simulink model "OnBoardOk"  (R2015b)
settings: Solver=FixedStepDiscrete  SolverMode=SingleTasking  StartTime=0.0  StopTime=10.0  FixedStep=0.002  RelTol=1e-3
PreLoadFcn:
  | waijung.modelPreload; % Required for working with Waijung Blockset. Do not remove.
undefined symbols (not defined in the file): CPHA_1Edge, CPOL_Low, Duplex, FirstBit_MSB, Full, Link, LQFP100, ST, STM32F407VG, STM32F4DISCOVERY
libraries: simulink x12, stm32f4_io_lib x5, stm32f4_spi_lib x3, stm32f4_device_config_lib x1, BC_USB x1, stm32f4_adc_lib x1
(part 1 of 2)
CloseFcn:
  | waijung.modelClose; % Required for working with Waijung Blockset. Do not remove.
settings Model: Creator=Hi  LastModifiedBy=Jasper Gundersen
settings DataIOCC: SaveFormat=Array
settings OptimizationCC: OptimizeModelRefInitCode=on  LifeSpan=1
settings HardwareCC: ProdBitPerPointer=32  ProdLargestAtomicFloat=None  ProdIntDivRoundTo=Undefined  ProdWordSize=32  ProdHWDeviceType=ARM Compatible->Cortex - M4  TargetEndianess=LittleEndian  TargetHWDeviceType=ARM Compatible->Cortex - M4
settings RTWCC: SystemTargetFile=stm32f4.tlc  GenerateMakefile=off  TemplateMakefile=ert_default_tmf  Description=STM32F4 Target
settings CodeAppCC: ForceParamTrailComments=on  IgnoreCustomStorageClasses=off  OperatorAnnotations=on  SimulinkDataObjDesc=on  InsertBlockDesc=on  MATLABSourceComments=on
settings STFCustomTargetCC: ModelReferenceCompliant=off  ConcurrentExecutionCompliant=off  GeneratePreprocessorConditionals=Use local settings  CombineOutputUpdateFcns=on  ERTCustomFileBanners=on  SupportContinuousTime=off  SupportNonInlinedSFcns=off  MATLABClassNameForMDSCustomization=Simulink.SoftwareTarget.ERTCustomization  CPPClassGenCompliant=off  GRTInterface=off  SystemTargetFile=stm32f4.tlc
settings ERTTargetCC: ModelReferenceCompliant=off  ParMdlRefBuildCompliant=off  CompOptLevelCompliant=off  ConcurrentExecutionCompliant=off  ERTFirstTimeCompliant=off  ModelStepFunctionPrototypeControlCompliant=off  CPPClassGenCompliant=off  UseToolchainInfoCompliant=off  ERTSrcFileBannerTemplate=stm32f4_code_template.cgt  ERTHdrFileBannerTemplate=stm32f4_code_template.cgt  ERTDataSrcFileTemplate=stm32f4_code_template.cgt  ERTDataHdrFileTemplate=stm32f4_code_template.cgt  ERTCustomFileTemplate=stm32f4_file_process.tlc
settings ConfigComp: CovModelRefEnable=Off

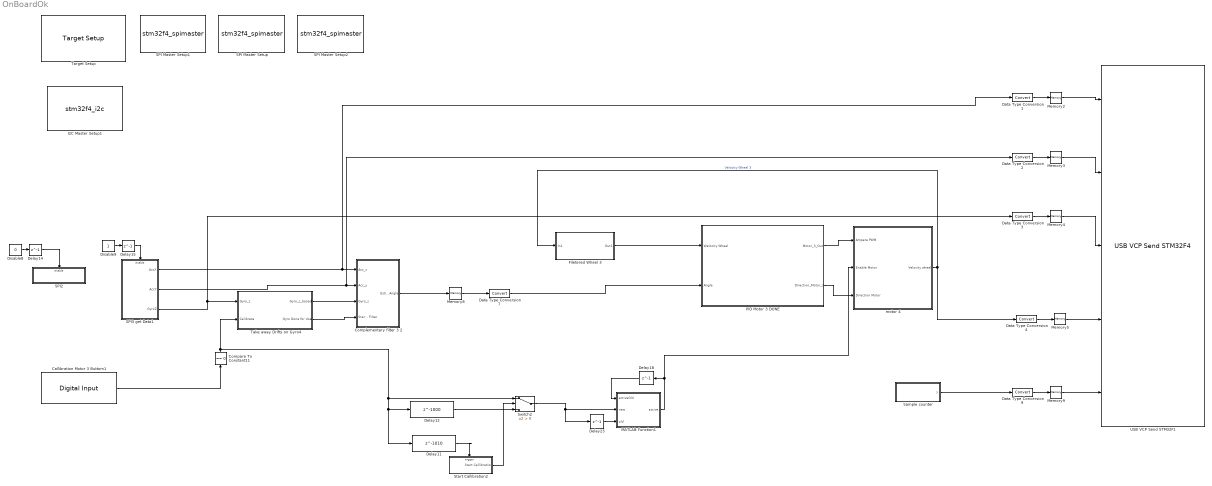
== system OnBoardOk ==
  Callibration Motor 3 Buttom1 : stm32f4_io_lib/Digital Input  port=E  speed=100  porttype=Pull Up  porttypestr=UP  use_pin0=off  use_pin1=off  use_pin2=off  use_pin3=off  use_pin4=off  use_pin5=off  use_pin6=off  use_pin7=off  use_pin8=off  use_pin9=off  use_pin10=on  use_pin11=off  use_pin12=off  use_pin13=off  use_pin14=off  use_pin15=off  pinstr=GPIO_Pin_10  usedpinarray="[0  0  0  0  0  0  0  0  0  0  1  0  0  0  0  0]"  bitbandingstr="#define CallibrationMotor3Buttom1_E10 Peripheral_BB(GPIOE->IDR, 10)  /* Output pin */"  sampletime=0.002  sampletimestr=0.002  blockid=CallibrationMotor3Buttom1  enablecustomportlabel=off  glabalinit=off  cinputportlabel=In1, In2  coutputportlabel=Out1, Out2
  Compare To Constant11 : simulink/Logic and Bit Operations/Compare To Constant  relop===  const=0  OutDataTypeStr=boolean  ZeroCross=off
  Complementary filter 3 2 : Subsystem
  Data Type Conversion{1..4,7,9} (6 alike) : DataTypeConversion
  Delay11 : Delay  DelayLength=1010  InitialCondition=0
  Delay12 : Delay  DelayLength=1000  InitialCondition=0
  Delay14 : Delay  DelayLength=1  InitialCondition=1
  Delay15 : Delay  DelayLength=1  InitialCondition=0
  Delay18 : Delay  DelayLength=1  InitialCondition=0
  Delay23 : Delay  DelayLength=1  InitialCondition=0
  Disable8 : Constant  Value=0
  Disable9 : Constant
  Filetered Wheel 3 : Subsystem
  I2C Master Setup1 : S-Function  FunctionName=stm32f4_i2c  Parameters=configuration,module,transfer,clkspeed,timeout,sdapin,sclpin,writecount,readcount,inputtypearray,outputtypearray,confstr,sampletime,sampletimestr,blockid  SFunctionDeploymentMode=off  EnableBusSupport=off  mask(stm32f4_i2c){configuration=Setup, module=1, lastmodule=1, transfer=Blocking, dutycycle=TLow/THigh = 2, clkspeed=400, timeout=25, writecount=0, readcount=0, sdapin=B7, sclpin=B6, waitwritetime=0, inputtypearray=[0], outputtypearray=[0], confstr=["B","7","B","6","1","1","6","0","I2C_DutyCycle_2","0","off"], sampletime=-1, sampletimestr=0.002, blockid=I2CMasterSetup1}
      mask prompts: module "I2C Module"; lastmodule "Last module"; transfer "Transfer mode"; dutycycle "Duty cycle in fast mode"; clkspeed "Clock speed (kHz)"; timeout "Timeout (ms)"; writecount "Bytes write count"; readcount "Bytes read count"; sdapin "SDA pin"; sclpin "SCL pin"; waitwritetime "Wait write time (ms), default is 0"; inputtypearray "Input type array"; outputtypearray "Output type array"; confstr "Configuration string"; sampletime "Sample time (sec)"; sampletimestr "Compiled sample time (sec) in string"
      mask init:
      | stm32f4_i2c_callback('init');
      mask Help: web(fullfile(waijungdocroot,'stm32f4_i2c_setup.htm'), '-browser')
      mask TypeOptions configuration: Setup | Transaction
      mask Callback configuration: stm32f4_i2c_callback('configuration');
      mask TypeOptions module: 1 | 2 | 3
      mask Callback module: stm32f4_i2c_callback('module');
      mask TypeOptions transfer: Blocking | Non-blocking
      mask TypeOptions dutycycle: TLow/THigh = 16/9 | TLow/THigh = 2
      mask Callback dutycycle: stm32f4_i2c_callback('dutycycle');
      mask Callback writecount: stm32f4_i2c_callback('writecount');
      mask Callback readcount: stm32f4_i2c_callback('readcount');
      mask TypeOptions sdapin: - | B7 | B9
      mask Callback sdapin: stm32f4_i2c_callback('sdapin');
      mask TypeOptions sclpin: - | B6 | B8
      mask Callback sclpin: stm32f4_i2c_callback('sclpin');
      mask Callback confstr: stm32f4_i2c_callback('confstr');
      mask Callback sampletime: stm32f4_i2c_callback('sampletime');
      mask Callback sampletimestr: stm32f4_i2c_callback('sampletimestr');
      mask Callback blockid: stm32f4_i2c_callback('blockid');
      mask Display: text(0.5, 0.5, 'Module: I2C1\nClock: 400kHz\nSDA/SCL Pin: B7/B6','ver','middle','hor','center');
  MATLAB Function1 : MATLAB Function  TreatAsAtomicUnit=on
  Memory{2..5,8..9} (6 alike) : Memory  InheritSampleTime=on
  "PID Motor 3 DONE " : Subsystem
  SPI Master Setup : S-Function  FunctionName=stm32f4_spimaster  Parameters=mode,configuration,module,datacount,inputtypearray,outputtypearray,confstr,sampletime,sampletimestr,blockid  SFunctionDeploymentMode=off  EnableBusSupport=off  mask(stm32f4_spimaster){configuration=Setup, module=2, mode=Write, lastmodule=2, direction=Full-Duplex, dataformat=8bit/ FirstBit_MSB, prescaler=32, lastpclk=42000000, baudrate=1312500, cpolcpha=CPOL_Low/ CPHA_1Edge, datacount=0, nssmode=Software, nsspin=Not used, softnssport=B, softnsspin=12, sckpin=B13, misopin=B14, mosipin=B15, pintype=Push Pull, pulltype=Pull Up, nssdelay=0, inputtypearray=[0], outputtypearray=[0], confstr=["SPI_Direction_2Lines_FullDuplex","8b","MSB","Low","1Edge","32","Soft","0","x","x","1","B","12","1","B","13","1","B","14","1","B","15","0","1","0","0","0","0","0","0","0","PP","0","UP"], sampletime=-1, sampletimestr=0.002, blockid=SPIMasterSetup}
      mask prompts: module "SPI Module:"; lastmodule "Last module:"; dataformat "Data format:"; prescaler "Buad rate prescaler: Pclk/"; lastpclk "Last PCLK"; baudrate "Baud rate (Hz)"; cpolcpha "Clock polarity (CPOL)/ Clock phase (CPHA):"; datacount "Data Write count:"; nssmode "Slave/chip select (nSS, nCS) mode"; nsspin "Slave/chip select (nSS, nCS) pin"; softnssport "Slave/chip select port (nSS, nCS)"; softnsspin "Slave/chip select pin (nSS, nCS)"; sckpin "SCLK pin:"; misopin "MISO pin:"; mosipin "MOSI pin:"; pintype "Pin type (Push-Pull/Open-Drain)"; pulltype "Pull Type (Up/Down)"; nssdelay "Data delay time, uS:"; inputtypearray "Input type array"; outputtypearray "Output type array"; confstr "Configuration string"; sampletime "Sample time (sec)"; sampletimestr "Compiled sample time (sec) in string"
      mask help:
      | Direction:
      |  - Full-Duplex, use this mode when need to send and receive data at same clock.
      |  - Half-Duplex_Tx, this mode is to transmit data to slave only. Pin MISO (Rx) can be free for other function.
      |  - Half-Duplex_Rx, this mode is to receive data from slave only. Pin MOSIO (Tx) can be free for other function.
      | Data format:
      |   This configuration is depending on the specification of slave device.
      | Baud rate prescaler:
      |  - Use this prescaler to devide from the PCLK for SPI clock.
      |  - This Prescaler value is auto determine corresponding to baudrate setting and selected SPI module.
      | Baud rate (Hz):
      |  - Select baud rate for SPI clock. Please check the maximum clock support for target slave device.
      | Clock polarity and Clock phase:
      |  - This configuration parameter is depending on slave device.
      |  - See waijung help for more description.
      | Slave/chip select mode:
      |  - Hardware, use hardware SPI module for slave select (or chip select) pin.
      |  - Software, this mode allow any available pin for slave select (or chip select) function.
      |  - Custom, SPI block did not control slave select pin. User may use Digital Output block to control by costom.
      mask init:
      | stm32f4_spimaster_callback('init');
      mask Help: web(fullfile(waijungdocroot,'stm32f4_spimaster_setup.htm'), '-browser')
      mask TypeOptions configuration: Setup | Transaction
      mask Callback configuration: stm32f4_spimaster_callback('configuration');
      mask TypeOptions module: 1 | 2 | 3
      mask Callback module: stm32f4_spimaster_callback('module');
      mask TypeOptions mode: Read/ Write | Read | Write
      mask Callback mode: stm32f4_spimaster_callback('mode');
      mask TypeOptions direction: Full-Duplex | Half-Duplex_Tx | Half-Duplex_Rx
      mask Callback direction: stm32f4_spimaster_callback('direction');
      mask TypeOptions dataformat: 8bit/ FirstBit_MSB | 8bit/ FirstBit_LSB | 16bit/ FirstBit_MSB | 16bit/ FirstBit_LSB
      mask TypeOptions prescaler: 2 | 4 | 8 | 16 | 32 | 64 | 128 | 256
      mask TypeOptions baudrate: Not set | 21000000 | 10500000 | 5250000 | 2625000 | 1312500 | 656250 | 328125 | 164063
      mask Callback baudrate: stm32f4_spimaster_callback('baudrate');
      mask TypeOptions cpolcpha: CPOL_Low/ CPHA_1Edge | CPOL_Low/ CPHA_2Edge | CPOL_High/ CPHA_1Edge | CPOL_High/ CPHA_2Edge
      mask Callback datacount: stm32f4_spimaster_callback('datacount');
      mask TypeOptions nssmode: Hardware | Software | Custom
      mask Callback nssmode: stm32f4_spimaster_callback('nssmode');
      mask TypeOptions nsspin: Not used | B9 | B12
      mask TypeOptions softnssport: A | B | C | D | E | F | G | H | I
      mask TypeOptions softnsspin: 0 | 1 | 2 | 3 | 4 | 5 | 6 | 7 | 8 | 9 | 10 | 11 | 12 | 13 | 14 | 15
      mask TypeOptions sckpin: Not used | B10 | B13
      mask TypeOptions misopin: Not used | B14 | C2
      mask TypeOptions mosipin: Not used | B15 | C3
      mask TypeOptions pintype: Push Pull | Open Drain
      mask TypeOptions pulltype: None | Pull Up | Pull Down
      mask Callback confstr: stm32f4_spimaster_callback('confstr');
      mask Callback sampletime: stm32f4_spimaster_callback('sampletime');
      mask Callback sampletimestr: stm32f4_spimaster_callback('sampletimestr');
      mask Callback blockid: stm32f4_spimaster_callback('blockid');
      mask Display: text(0.5, 0.5, 'Module: SPI2 (Master)\nFull-Duplex\nBaudrate: 1312500','ver','middle','hor','center');
  SPI Master Setup1 : S-Function  FunctionName=stm32f4_spimaster  Parameters=mode,configuration,module,datacount,inputtypearray,outputtypearray,confstr,sampletime,sampletimestr,blockid  SFunctionDeploymentMode=off  EnableBusSupport=off  mask(stm32f4_spimaster){configuration=Setup, module=1, mode=Write, lastmodule=1, direction=Full-Duplex, dataformat=8bit/ FirstBit_MSB, prescaler=64, lastpclk=84000000, baudrate=1312500, cpolcpha=CPOL_Low/ CPHA_1Edge, datacount=0, nssmode=Software, nsspin=Not used, softnssport=C, softnsspin=5, sckpin=A5, misopin=A6, mosipin=A7, pintype=Push Pull, pulltype=Pull Up, nssdelay=0, inputtypearray=[0], outputtypearray=[0], confstr=["SPI_Direction_2Lines_FullDuplex","8b","MSB","Low","1Edge","64","Soft","0","x","x","1","C","5","1","A","5","1","A","6","1","A","7","1","0","1","0","0","0","0","0","0","PP","0","UP"], sampletime=-1, sampletimestr=0.002, blockid=SPIMasterSetup1}
      mask prompts: module "SPI Module:"; lastmodule "Last module:"; dataformat "Data format:"; prescaler "Buad rate prescaler: Pclk/"; lastpclk "Last PCLK"; baudrate "Baud rate (Hz)"; cpolcpha "Clock polarity (CPOL)/ Clock phase (CPHA):"; datacount "Data Write count:"; nssmode "Slave/chip select (nSS, nCS) mode"; nsspin "Slave/chip select (nSS, nCS) pin"; softnssport "Slave/chip select port (nSS, nCS)"; softnsspin "Slave/chip select pin (nSS, nCS)"; sckpin "SCLK pin:"; misopin "MISO pin:"; mosipin "MOSI pin:"; pintype "Pin type (Push-Pull/Open-Drain)"; pulltype "Pull Type (Up/Down)"; nssdelay "Data delay time, uS:"; inputtypearray "Input type array"; outputtypearray "Output type array"; confstr "Configuration string"; sampletime "Sample time (sec)"; sampletimestr "Compiled sample time (sec) in string"
      mask help:
      | Direction:
      |  - Full-Duplex, use this mode when need to send and receive data at same clock.
      |  - Half-Duplex_Tx, this mode is to transmit data to slave only. Pin MISO (Rx) can be free for other function.
      |  - Half-Duplex_Rx, this mode is to receive data from slave only. Pin MOSIO (Tx) can be free for other function.
      | Data format:
      |   This configuration is depending on the specification of slave device.
      | Baud rate prescaler:
      |  - Use this prescaler to devide from the PCLK for SPI clock.
      |  - This Prescaler value is auto determine corresponding to baudrate setting and selected SPI module.
      | Baud rate (Hz):
      |  - Select baud rate for SPI clock. Please check the maximum clock support for target slave device.
      | Clock polarity and Clock phase:
      |  - This configuration parameter is depending on slave device.
      |  - See waijung help for more description.
      | Slave/chip select mode:
      |  - Hardware, use hardware SPI module for slave select (or chip select) pin.
      |  - Software, this mode allow any available pin for slave select (or chip select) function.
      |  - Custom, SPI block did not control slave select pin. User may use Digital Output block to control by costom.
      mask init:
      | stm32f4_spimaster_callback('init');
      mask Help: web(fullfile(waijungdocroot,'stm32f4_spimaster_setup.htm'), '-browser')
      mask TypeOptions configuration: Setup | Transaction
      mask Callback configuration: stm32f4_spimaster_callback('configuration');
      mask TypeOptions module: 1 | 2 | 3
      mask Callback module: stm32f4_spimaster_callback('module');
      mask TypeOptions mode: Read/ Write | Read | Write
      mask Callback mode: stm32f4_spimaster_callback('mode');
      mask TypeOptions direction: Full-Duplex | Half-Duplex_Tx | Half-Duplex_Rx
      mask Callback direction: stm32f4_spimaster_callback('direction');
      mask TypeOptions dataformat: 8bit/ FirstBit_MSB | 8bit/ FirstBit_LSB | 16bit/ FirstBit_MSB | 16bit/ FirstBit_LSB
      mask TypeOptions prescaler: 2 | 4 | 8 | 16 | 32 | 64 | 128 | 256
      mask TypeOptions baudrate: Not set | 42000000 | 21000000 | 10500000 | 5250000 | 2625000 | 1312500 | 656250 | 328125
      mask Callback baudrate: stm32f4_spimaster_callback('baudrate');
      mask TypeOptions cpolcpha: CPOL_Low/ CPHA_1Edge | CPOL_Low/ CPHA_2Edge | CPOL_High/ CPHA_1Edge | CPOL_High/ CPHA_2Edge
      mask Callback datacount: stm32f4_spimaster_callback('datacount');
      mask TypeOptions nssmode: Hardware | Software | Custom
      mask Callback nssmode: stm32f4_spimaster_callback('nssmode');
      mask TypeOptions nsspin: Not used | A4 | A15
      mask TypeOptions softnssport: A | B | C | D | E | F | G | H | I
      mask TypeOptions softnsspin: 0 | 1 | 2 | 3 | 4 | 5 | 6 | 7 | 8 | 9 | 10 | 11 | 12 | 13 | 14 | 15
      mask TypeOptions sckpin: Not used | A5 | B3
      mask TypeOptions misopin: Not used | A6 | B4
      mask TypeOptions mosipin: Not used | A7 | B5
      mask TypeOptions pintype: Push Pull | Open Drain
      mask TypeOptions pulltype: None | Pull Up | Pull Down
      mask Callback confstr: stm32f4_spimaster_callback('confstr');
      mask Callback sampletime: stm32f4_spimaster_callback('sampletime');
      mask Callback sampletimestr: stm32f4_spimaster_callback('sampletimestr');
      mask Callback blockid: stm32f4_spimaster_callback('blockid');
      mask Display: text(0.5, 0.5, 'Module: SPI1 (Master)\nFull-Duplex\nBaudrate: 1312500','ver','middle','hor','center');
  SPI Master Setup2 : S-Function  FunctionName=stm32f4_spimaster  Parameters=mode,configuration,module,datacount,inputtypearray,outputtypearray,confstr,sampletime,sampletimestr,blockid  SFunctionDeploymentMode=off  EnableBusSupport=off  mask(stm32f4_spimaster){configuration=Setup, module=3, mode=Write, lastmodule=3, direction=Full-Duplex, dataformat=8bit/ FirstBit_MSB, prescaler=32, lastpclk=42000000, baudrate=1312500, cpolcpha=CPOL_Low/ CPHA_1Edge, datacount=0, nssmode=Software, nsspin=Not used, softnssport=C, softnsspin=11, sckpin=C10, misopin=B4, mosipin=B5, pintype=Push Pull, pulltype=Pull Up, nssdelay=0, inputtypearray=[0], outputtypearray=[0], confstr=["SPI_Direction_2Lines_FullDuplex","8b","MSB","Low","1Edge","32","Soft","0","x","x","1","C","11","1","C","10","1","B","4","1","B","5","0","1","1","0","0","0","0","0","0","PP","0","UP"], sampletime=-1, sampletimestr=0.002, blockid=SPIMasterSetup2}
      mask prompts: module "SPI Module:"; lastmodule "Last module:"; dataformat "Data format:"; prescaler "Buad rate prescaler: Pclk/"; lastpclk "Last PCLK"; baudrate "Baud rate (Hz)"; cpolcpha "Clock polarity (CPOL)/ Clock phase (CPHA):"; datacount "Data Write count:"; nssmode "Slave/chip select (nSS, nCS) mode"; nsspin "Slave/chip select (nSS, nCS) pin"; softnssport "Slave/chip select port (nSS, nCS)"; softnsspin "Slave/chip select pin (nSS, nCS)"; sckpin "SCLK pin:"; misopin "MISO pin:"; mosipin "MOSI pin:"; pintype "Pin type (Push-Pull/Open-Drain)"; pulltype "Pull Type (Up/Down)"; nssdelay "Data delay time, uS:"; inputtypearray "Input type array"; outputtypearray "Output type array"; confstr "Configuration string"; sampletime "Sample time (sec)"; sampletimestr "Compiled sample time (sec) in string"
      mask help:
      | Direction:
      |  - Full-Duplex, use this mode when need to send and receive data at same clock.
      |  - Half-Duplex_Tx, this mode is to transmit data to slave only. Pin MISO (Rx) can be free for other function.
      |  - Half-Duplex_Rx, this mode is to receive data from slave only. Pin MOSIO (Tx) can be free for other function.
      | Data format:
      |   This configuration is depending on the specification of slave device.
      | Baud rate prescaler:
      |  - Use this prescaler to devide from the PCLK for SPI clock.
      |  - This Prescaler value is auto determine corresponding to baudrate setting and selected SPI module.
      | Baud rate (Hz):
      |  - Select baud rate for SPI clock. Please check the maximum clock support for target slave device.
      | Clock polarity and Clock phase:
      |  - This configuration parameter is depending on slave device.
      |  - See waijung help for more description.
      | Slave/chip select mode:
      |  - Hardware, use hardware SPI module for slave select (or chip select) pin.
      |  - Software, this mode allow any available pin for slave select (or chip select) function.
      |  - Custom, SPI block did not control slave select pin. User may use Digital Output block to control by costom.
      mask init:
      | stm32f4_spimaster_callback('init');
      mask Help: web(fullfile(waijungdocroot,'stm32f4_spimaster_setup.htm'), '-browser')
      mask TypeOptions configuration: Setup | Transaction
      mask Callback configuration: stm32f4_spimaster_callback('configuration');
      mask TypeOptions module: 1 | 2 | 3
      mask Callback module: stm32f4_spimaster_callback('module');
      mask TypeOptions mode: Read/ Write | Read | Write
      mask Callback mode: stm32f4_spimaster_callback('mode');
      mask TypeOptions direction: Full-Duplex | Half-Duplex_Tx | Half-Duplex_Rx
      mask Callback direction: stm32f4_spimaster_callback('direction');
      mask TypeOptions dataformat: 8bit/ FirstBit_MSB | 8bit/ FirstBit_LSB | 16bit/ FirstBit_MSB | 16bit/ FirstBit_LSB
      mask TypeOptions prescaler: 2 | 4 | 8 | 16 | 32 | 64 | 128 | 256
      mask TypeOptions baudrate: Not set | 21000000 | 10500000 | 5250000 | 2625000 | 1312500 | 656250 | 328125 | 164063
      mask Callback baudrate: stm32f4_spimaster_callback('baudrate');
      mask TypeOptions cpolcpha: CPOL_Low/ CPHA_1Edge | CPOL_Low/ CPHA_2Edge | CPOL_High/ CPHA_1Edge | CPOL_High/ CPHA_2Edge
      mask Callback datacount: stm32f4_spimaster_callback('datacount');
      mask TypeOptions nssmode: Hardware | Software | Custom
      mask Callback nssmode: stm32f4_spimaster_callback('nssmode');
      mask TypeOptions nsspin: Not used | A4 | A15
      mask TypeOptions softnssport: A | B | C | D | E | F | G | H | I
      mask TypeOptions softnsspin: 0 | 1 | 2 | 3 | 4 | 5 | 6 | 7 | 8 | 9 | 10 | 11 | 12 | 13 | 14 | 15
      mask TypeOptions sckpin: Not used | B3 | C10
      mask TypeOptions misopin: Not used | B4 | C11
      mask TypeOptions mosipin: Not used | B5 | C12
      mask TypeOptions pintype: Push Pull | Open Drain
      mask TypeOptions pulltype: None | Pull Up | Pull Down
      mask Callback confstr: stm32f4_spimaster_callback('confstr');
      mask Callback sampletime: stm32f4_spimaster_callback('sampletime');
      mask Callback sampletimestr: stm32f4_spimaster_callback('sampletimestr');
      mask Callback blockid: stm32f4_spimaster_callback('blockid');
      mask Display: text(0.5, 0.5, 'Module: SPI3 (Master)\nFull-Duplex\nBaudrate: 1312500','ver','middle','hor','center');
  SPI2 : Subsystem  Priority=0  TreatAsAtomicUnit=on
  SPI3 get Data1 : Subsystem
  Sample counter : MATLAB Function  TreatAsAtomicUnit=on
  Start Callibration2 : Subsystem
  Switch2 : Switch  Criteria=u2 > Threshold
  Take away Drifts on Gyro4 : Subsystem
  Target Setup : stm32f4_device_config_lib/Target Setup  Priority=100  compiler=GNU ARM  previous_compiler=GNU ARM  mcu=STM32F407VG (LQFP100); STM32F4DISCOVERY  mcustr=STM32F407VG  clockconfig=STM32F4DISCOVERY Default (HSEOSC-8MHz/HCLK-168MHz)  system_stm32f4xx_c_path=C:\Users\Jasper Gundersen\Documents\Cube\waijung15_04a\targets\stm32f4_target\stm32f4\utils\STM32F4xx_AN3988_V1.0.1\stm32f4_default\hseosc8mhz  showmemoryconfiguration=off  stacksize=0x400  heapsize=0x200  enableautocompiledownload=on  fullchiperase=off  programmerinterface=ST-Link  editctrlstr=on  compilercontrolstr=$(patsubst %, -I%, .) -mcpu=cortex-m4 -mthumb -mthumb-interwork -mfloat-abi=hard -mfpu=fpv4-sp-d16 -ffast-math -Wall -Wextra -Ofast  assemblercontrolstr=$(patsubst %, -I%, .) -mcpu=cortex-m4 -mthumb -mthumb-interwork -mfloat-abi=hard -mfpu=fpv4-sp-d16 -ffast-math -Wall -Wextra -Ofast -Wa,-amhls=$(<:.s=.lst) -D__STACK_SIZE=$(STACK_SIZE) -D__HEAP_SIZE=$(HEAP_SIZE)  linkercontrolstr=-T$(LD_SCRIPT) -g -Wl,-Map=$(MAP),--cref,--no-warn-mismatch -mcpu=cortex-m4 -mthumb -mthumb-interwork -mfloat-abi=hard -mfpu=fpv4-sp-d16  runafterdownload=on  execprofile=None  profileruart=1  profilerbaud=115200  profilertxpin=Not used  profilerinitstr=0.002,168000000,336000,115200,0  manualsetsampletime=on  sampletime=0.002  blockid=TargetSetup  systickreloadvalue=336000  hseval=8000000  lastprofileruart=1  hclk=168000000  flashorigin=0x8000000  flashlength=1M  ramorigin=0x20000000  ramlength=112k  useextram=off
  USB VCP Send STM32F1 : BC_USB/USB VCP Send STM32F4  speed="USB 1.1   12Mbit/s"  data_size=2048 Bytes  header_data='0E 0E'  binary_data='double double double double double'  terminator_data='0A 0A'  sampletime=0.002
  motor 4 : Subsystem
  wires:
  Delay14/1 -> SPI2/Enable
  Disable8/1 -> Delay14/1
  Disable9/1 -> Delay15/1
  Delay15/1 -> SPI3 get Data1/Enable
  Callibration Motor 3 Buttom1/1 -> Compare To Constant11/1
  Take away Drifts on Gyro4/1(Gyro_z_based) -> Complementary filter 3 2/3(Gyro_z)
  Take away Drifts on Gyro4/2(Gyro Done for Use) -> Complementary filter 3 2/4("Start Complementary Filter ")
  SPI3 get Data1/1(AccX) -> Data Type Conversion1/1, Complementary filter 3 2/1(Acc_x)
  SPI3 get Data1/2("AccY ") -> Data Type Conversion2/1, Complementary filter 3 2/2(Acc_y)
  SPI3 get Data1/3(GyroZ) -> Data Type Conversion3/1, Take away Drifts on Gyro4/1(Gyro_z)
  motor 4/1(Velocity wheel) -> Filetered Wheel 3/1(In1), Data Type Conversion4/1  "Velocity Wheel 3"
  Filetered Wheel 3/1(Out1) -> "PID Motor 3 DONE "/1("Welocity Wheel ")
  Data Type Conversion7/1 -> "PID Motor 3 DONE "/2(Angle)
  "PID Motor 3 DONE "/1(Motor_3_Out) -> motor 4/1(Ampere PWM)
  Complementary filter 3 2/1(Estimated_Angle) -> Memory8/1
  Memory8/1 -> Data Type Conversion7/1
  Compare To Constant11/1 -> Switch2/1, Delay11/1, Delay12/1, Take away Drifts on Gyro4/2(Calibrate)
  MATLAB Function1/1(active) -> motor 4/2(Enable Motor), Delay18/1
  Delay23/1 -> MATLAB Function1/3(old)
  Switch2/1 -> Delay23/1, MATLAB Function1/2(new)
  Delay18/1 -> MATLAB Function1/1(activeOld)
  Start Callibration2/1(Start Callibration) -> Switch2/2
  Delay11/1 -> Start Callibration2/Trigger
  Delay12/1 -> Switch2/3
  Data Type Conversion1/1 -> Memory2/1
  Memory2/1 -> USB VCP Send STM32F1/1
  Data Type Conversion2/1 -> Memory3/1
  Memory3/1 -> USB VCP Send STM32F1/2
  Data Type Conversion3/1 -> Memory4/1
  Memory4/1 -> USB VCP Send STM32F1/3
  Data Type Conversion4/1 -> Memory5/1
  Memory5/1 -> USB VCP Send STM32F1/4
  Data Type Conversion9/1 -> Memory9/1
  "PID Motor 3 DONE "/2("Direction_Motor_3 ") -> motor 4/3("Direction Motor ")
  Sample counter/1(y) -> Data Type Conversion9/1
  Memory9/1 -> USB VCP Send STM32F1/5

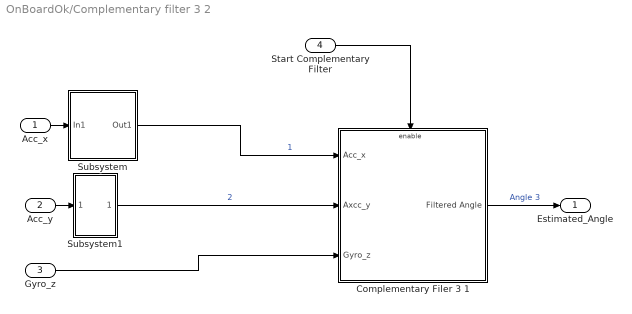
== system OnBoardOk/Complementary filter 3 2 ==
  Acc_x : Inport
  Acc_y : Inport  Port=2
  Gyro_z : Inport  Port=3
  "Start Complementary Filter " : Inport  Port=4
  Complementary Filer 3 1 : Subsystem
  Subsystem : Subsystem
  Subsystem1 : Subsystem
  Estimated_Angle : Outport
  wires:
  Subsystem/1(Out1) -> Complementary Filer 3 1/1(Acc_x)  "1"
  Subsystem1/1(Out1) -> Complementary Filer 3 1/2(Axcc_y)  "2"
  Gyro_z/1 -> Complementary Filer 3 1/3(Gyro_z)
  "Start Complementary Filter "/1 -> Complementary Filer 3 1/Enable
  Complementary Filer 3 1/1(Filtered Angle) -> Estimated_Angle/1  "Angle 3"
  Acc_y/1 -> Subsystem1/1(In1)
  Acc_x/1 -> Subsystem/1(In1)

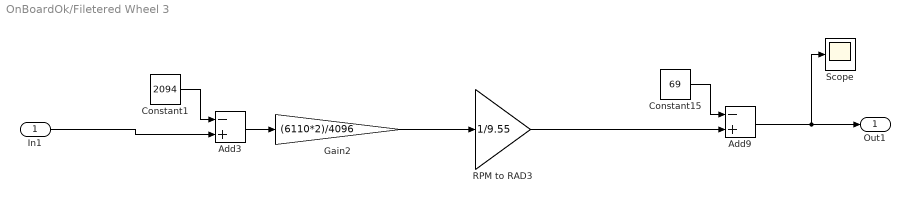
== system OnBoardOk/Filetered Wheel 3 ==
  In1 : Inport
  Add3 : Sum  Inputs=-+
  Add9 : Sum  Inputs=-+
  Constant1 : Constant  Value=2094  SampleTime=-1
  Constant15 : Constant  Value=69  SampleTime=-1
  Gain2 : Gain  Gain=(6110*2)/4096
  RPM to RAD3 : Gain  Gain=1/9.55
  Scope : Scope
  Out1 : Outport
  wires:
  Gain2/1 -> RPM to RAD3/1
  Add3/1 -> Gain2/1
  Constant1/1 -> Add3/1
  In1/1 -> Add3/2
  Constant15/1 -> Add9/1
  RPM to RAD3/1 -> Add9/2
  Add9/1 -> Scope/1, Out1/1

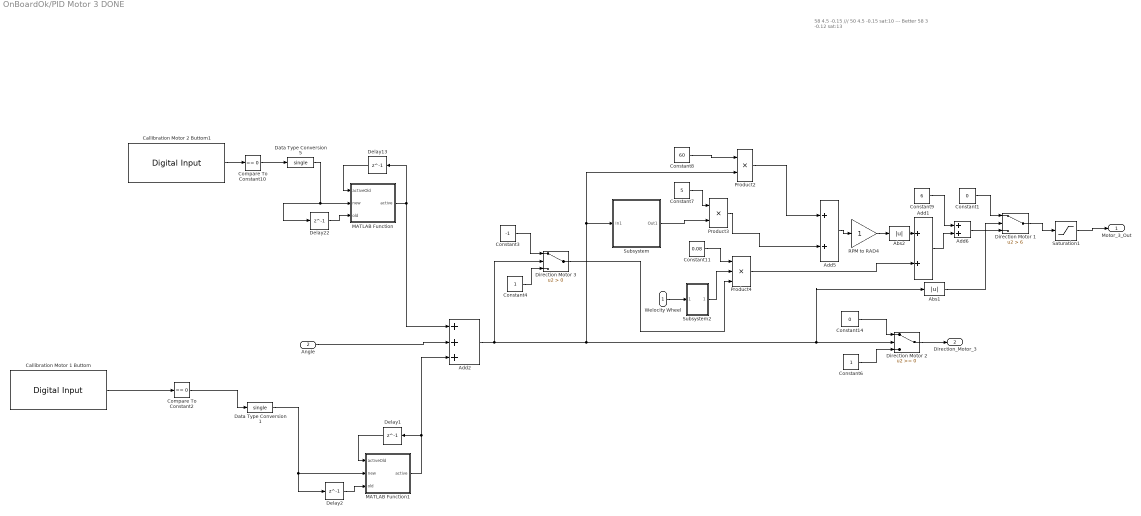
== system OnBoardOk/PID Motor 3 DONE  ==
  note: 58
      | 4.5
      | -0.15
      | ///
      | 50
      | 4.5
      | -0.15
      | sat:10
      | --- Better
      | 58
      | 3
      | -0.12
      | sat:13
  "Welocity Wheel " : Inport
  Angle : Inport  Port=2
  Abs1 : Abs
  Abs2 : Abs
  Add1 : Sum
  Add2 : Sum  Inputs=+++
  Add5 : Sum
  Add6 : Sum
  Callibration Motor 1 Buttom : stm32f4_io_lib/Digital Input  port=E  speed=100  porttype=Pull Up  porttypestr=UP  use_pin0=off  use_pin1=off  use_pin2=off  use_pin3=off  use_pin4=off  use_pin5=off  use_pin6=off  use_pin7=off  use_pin8=off  use_pin9=off  use_pin10=off  use_pin11=off  use_pin12=off  use_pin13=off  use_pin14=on  use_pin15=off  pinstr=GPIO_Pin_14  usedpinarray="[0  0  0  0  0  0  0  0  0  0  0  0  0  0  1  0]"  bitbandingstr="#define PIDMotor3DONECallibrationMotor1Buttom_E14 Peripheral_BB(GPIOE->IDR, 14)  /* Output pin */"  sampletime=0.002  sampletimestr=0.002  blockid=PIDMotor3DONECallibrationMotor1Buttom  enablecustomportlabel=off  glabalinit=off  cinputportlabel=In1, In2  coutputportlabel=Out1, Out2
  Callibration Motor 2 Buttom1 : stm32f4_io_lib/Digital Input  port=E  speed=100  porttype=Pull Up  porttypestr=UP  use_pin0=off  use_pin1=off  use_pin2=off  use_pin3=off  use_pin4=off  use_pin5=off  use_pin6=off  use_pin7=off  use_pin8=off  use_pin9=off  use_pin10=off  use_pin11=on  use_pin12=off  use_pin13=off  use_pin14=off  use_pin15=off  pinstr=GPIO_Pin_11  usedpinarray="[0  0  0  0  0  0  0  0  0  0  0  1  0  0  0  0]"  bitbandingstr="#define PIDMotor3DONECallibrationMotor2Buttom1_E11 Peripheral_BB(GPIOE->IDR, 11)  /* Output pin */"  sampletime=0.002  sampletimestr=0.002  blockid=PIDMotor3DONECallibrationMotor2Buttom1  enablecustomportlabel=off  glabalinit=off  cinputportlabel=In1, In2  coutputportlabel=Out1, Out2
  Compare To Constant10 : simulink/Logic and Bit Operations/Compare To Constant  relop===  const=0  OutDataTypeStr=boolean  ZeroCross=off
  Compare To Constant2 : simulink/Logic and Bit Operations/Compare To Constant  relop===  const=0  OutDataTypeStr=boolean  ZeroCross=off
  Constant1 : Constant  Value=0  OutDataTypeStr=single  SampleTime=-1
  Constant11 : Constant  Value=0.08  OutDataTypeStr=single  SampleTime=-1
  Constant14 : Constant  Value=0  OutDataTypeStr=single  SampleTime=-1
  Constant3 : Constant  Value=-1  OutDataTypeStr=single  SampleTime=-1
  Constant4 : Constant  OutDataTypeStr=single  SampleTime=-1
  Constant6 : Constant  OutDataTypeStr=single  SampleTime=-1
  Constant7 : Constant  Value=5  OutDataTypeStr=single  SampleTime=-1
  Constant8 : Constant  Value=60  OutDataTypeStr=single  SampleTime=-1
  Constant9 : Constant  Value=6  SampleTime=-1
  Data Type Conversion1 : DataTypeConversion  OutDataTypeStr=single
  Data Type Conversion5 : DataTypeConversion  OutDataTypeStr=single
  Delay{1..2,13,22} (4 alike) : Delay  DelayLength=1  InitialCondition=0
  Direction Motor 1 : Switch  Criteria=u2 > Threshold  Threshold=6
  Direction Motor 2 : Switch
  Direction Motor 3 : Switch  Criteria=u2 > Threshold
  MATLAB Function : MATLAB Function  TreatAsAtomicUnit=on
  MATLAB Function1 : MATLAB Function  TreatAsAtomicUnit=on
  Product2 : Product
  Product3 : Product
  Product4 : Product  Inputs=3
  RPM to RAD4 : Gain
  Saturation1 : Saturate  UpperLimit=90  LowerLimit=10
  Subsystem : Subsystem
  Subsystem2 : Subsystem
  Motor_3_Out : Outport
  "Direction_Motor_3 " : Outport  Port=2
  wires:
  Direction Motor 2/1 -> "Direction_Motor_3 "/1
  Constant7/1 -> Product3/1
  Constant11/1 -> Product4/1
  Constant14/1 -> Direction Motor 2/1
  Constant6/1 -> Direction Motor 2/3
  Product3/1 -> Add5/2
  Constant9/1 -> Add6/1
  Add5/1 -> RPM to RAD4/1
  RPM to RAD4/1 -> Abs2/1
  Product2/1 -> Add5/1
  Abs2/1 -> Add1/1
  Saturation1/1 -> Motor_3_Out/1
  Constant8/1 -> Product2/1
  Add6/1 -> Direction Motor 1/3
  Direction Motor 1/1 -> Saturation1/1
  Constant1/1 -> Direction Motor 1/1
  Abs1/1 -> Direction Motor 1/2
  Product4/1 -> Add1/2
  "Welocity Wheel "/1 -> Subsystem2/1(In1)
  Angle/1 -> Add2/2
  Subsystem/1(Out1) -> Product3/2
  Add1/1 -> Add6/2
  Constant4/1 -> Direction Motor 3/3
  Constant3/1 -> Direction Motor 3/1
  Direction Motor 3/1 -> Product4/3
  Subsystem2/1(Out2) -> Product4/2
  Add2/1 -> Direction Motor 3/2, Subsystem/1(In1), Product2/2, Abs1/1, Direction Motor 2/2
  Callibration Motor 2 Buttom1/1 -> Compare To Constant10/1
  Compare To Constant10/1 -> Data Type Conversion5/1
  Callibration Motor 1 Buttom/1 -> Compare To Constant2/1
  Compare To Constant2/1 -> Data Type Conversion1/1
  MATLAB Function/1(active) -> Delay13/1, Add2/1
  Delay22/1 -> MATLAB Function/3(old)
  Data Type Conversion5/1 -> Delay22/1, MATLAB Function/2(new)
  Delay13/1 -> MATLAB Function/1(activeOld)
  MATLAB Function1/1(active) -> Add2/3, Delay1/1
  Delay2/1 -> MATLAB Function1/3(old)
  Data Type Conversion1/1 -> Delay2/1, MATLAB Function1/2(new)
  Delay1/1 -> MATLAB Function1/1(activeOld)

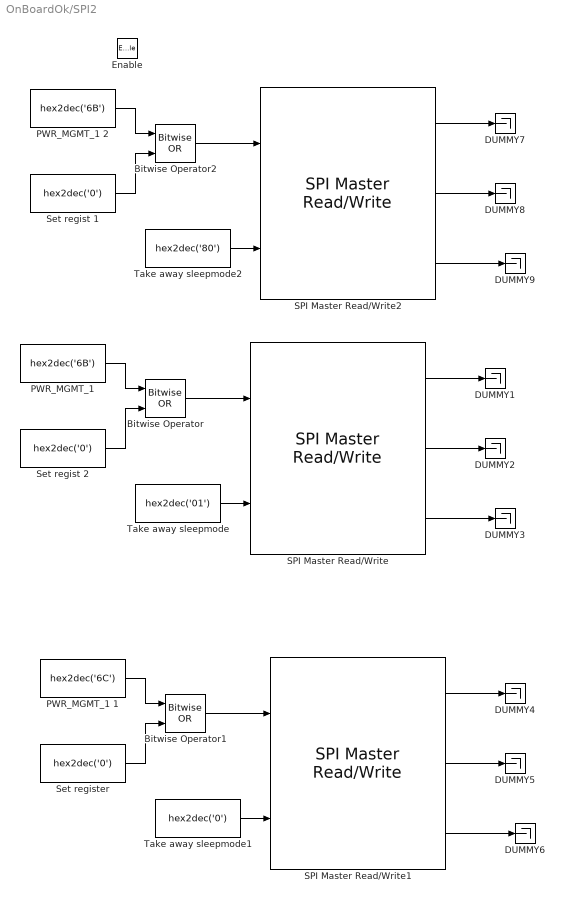
== system OnBoardOk/SPI2 ==
  Enable : EnablePort
  Bitwise Operator : simulink/Logic and Bit Operations/Bitwise Operator  logicop=OR  UseBitMask=off  NumInputPorts=2  BitMask=bin2dec('11011001')  BitMaskRealWorld=Stored Integer
  Bitwise Operator1 : simulink/Logic and Bit Operations/Bitwise Operator  logicop=OR  UseBitMask=off  NumInputPorts=2  BitMask=bin2dec('11011001')  BitMaskRealWorld=Stored Integer
  Bitwise Operator2 : simulink/Logic and Bit Operations/Bitwise Operator  logicop=OR  UseBitMask=off  NumInputPorts=2  BitMask=bin2dec('11011001')  BitMaskRealWorld=Stored Integer
  DUMMY{1..9} (9 alike) : Terminator
  "PWR_MGMT_1 " : Constant  Value=hex2dec('6B')  OutDataTypeStr=uint8
  PWR_MGMT_1 1 : Constant  Value=hex2dec('6C')  OutDataTypeStr=uint8
  PWR_MGMT_1 2 : Constant  Value=hex2dec('6B')  OutDataTypeStr=uint8
  SPI Master Read/Write : stm32f4_spi_lib/SPI Master Read//Write  configuration=Transaction  module=3  mode=Read/ Write  lastmodule=1  direction=Full-Duplex  dataformat=8bit/ FirstBit_MSB  prescaler=4  cpolcpha=CPOL_Low/ CPHA_1Edge  datacount=2  nssmode=Custom  nsspin=Not used  softnssport=E  softnsspin=0  sckpin=A5  misopin=A6  mosipin=A7  inputtypearray=[2 3 3]  outputtypearray=[3 7 3 3]  confstr="[\"SPI_Direction_2Lines_FullDuplex\",\"8b\",\"MSB\",\"Low\",\"1Edge\",\"4\",\"Soft\",\"0\",\"x\",\"x\",\"0\",\"x\",\"x\",\"1\",\"A\",\"5\",\"1\",\"A\",\"6\",\"1\",\"A\",\"7\",\"1\",\"0\",\"0\",\"0\",\"0\",\"0\",\"0\",\"0\",\"0\",\"PP\",\"0\",\"UP\"]"  sampletime=-1  sampletimestr=Inf  blockid=SPI2SPIMasterReadWrite
  SPI Master Read/Write1 : stm32f4_spi_lib/SPI Master Read//Write  configuration=Transaction  module=3  mode=Read/ Write  lastmodule=1  direction=Full-Duplex  dataformat=8bit/ FirstBit_MSB  prescaler=4  cpolcpha=CPOL_Low/ CPHA_1Edge  datacount=2  nssmode=Custom  nsspin=Not used  softnssport=E  softnsspin=0  sckpin=A5  misopin=A6  mosipin=A7  inputtypearray=[2 3 3]  outputtypearray=[3 7 3 3]  confstr="[\"SPI_Direction_2Lines_FullDuplex\",\"8b\",\"MSB\",\"Low\",\"1Edge\",\"4\",\"Soft\",\"0\",\"x\",\"x\",\"0\",\"x\",\"x\",\"1\",\"A\",\"5\",\"1\",\"A\",\"6\",\"1\",\"A\",\"7\",\"1\",\"0\",\"0\",\"0\",\"0\",\"0\",\"0\",\"0\",\"0\",\"PP\",\"0\",\"UP\"]"  sampletime=-1  sampletimestr=Inf  blockid=SPI2SPIMasterReadWrite1
  SPI Master Read/Write2 : stm32f4_spi_lib/SPI Master Read//Write  configuration=Transaction  module=3  mode=Read/ Write  lastmodule=1  direction=Full-Duplex  dataformat=8bit/ FirstBit_MSB  prescaler=4  cpolcpha=CPOL_Low/ CPHA_1Edge  datacount=2  nssmode=Custom  nsspin=Not used  softnssport=E  softnsspin=0  sckpin=A5  misopin=A6  mosipin=A7  inputtypearray=[2 3 3]  outputtypearray=[3 7 3 3]  confstr="[\"SPI_Direction_2Lines_FullDuplex\",\"8b\",\"MSB\",\"Low\",\"1Edge\",\"4\",\"Soft\",\"0\",\"x\",\"x\",\"0\",\"x\",\"x\",\"1\",\"A\",\"5\",\"1\",\"A\",\"6\",\"1\",\"A\",\"7\",\"1\",\"0\",\"0\",\"0\",\"0\",\"0\",\"0\",\"0\",\"0\",\"PP\",\"0\",\"UP\"]"  sampletime=-1  sampletimestr=Inf  blockid=SPI2SPIMasterReadWrite2
  Set regist 1 : Constant  Value=hex2dec('0')  OutDataTypeStr=uint8
  Set regist 2 : Constant  Value=hex2dec('0')  OutDataTypeStr=uint8
  Set register : Constant  Value=hex2dec('0')  OutDataTypeStr=uint8
  Take away sleepmode : Constant  Value=hex2dec('01')  OutDataTypeStr=uint8
  Take away sleepmode1 : Constant  Value=hex2dec('0')  OutDataTypeStr=uint8
  Take away sleepmode2 : Constant  Value=hex2dec('80')  OutDataTypeStr=uint8
  wires:
  SPI Master Read/Write/1 -> DUMMY1/1
  SPI Master Read/Write/2 -> DUMMY2/1
  SPI Master Read/Write/3 -> DUMMY3/1
  Bitwise Operator/1 -> SPI Master Read/Write/1
  Set regist 2/1 -> Bitwise Operator/2
  "PWR_MGMT_1 "/1 -> Bitwise Operator/1
  Take away sleepmode/1 -> SPI Master Read/Write/2
  SPI Master Read/Write1/1 -> DUMMY4/1
  SPI Master Read/Write1/2 -> DUMMY5/1
  SPI Master Read/Write1/3 -> DUMMY6/1
  Bitwise Operator1/1 -> SPI Master Read/Write1/1
  Set register/1 -> Bitwise Operator1/2
  PWR_MGMT_1 1/1 -> Bitwise Operator1/1
  Take away sleepmode1/1 -> SPI Master Read/Write1/2
  SPI Master Read/Write2/1 -> DUMMY7/1
  SPI Master Read/Write2/2 -> DUMMY8/1
  SPI Master Read/Write2/3 -> DUMMY9/1
  Bitwise Operator2/1 -> SPI Master Read/Write2/1
  Set regist 1/1 -> Bitwise Operator2/2
  PWR_MGMT_1 2/1 -> Bitwise Operator2/1
  Take away sleepmode2/1 -> SPI Master Read/Write2/2

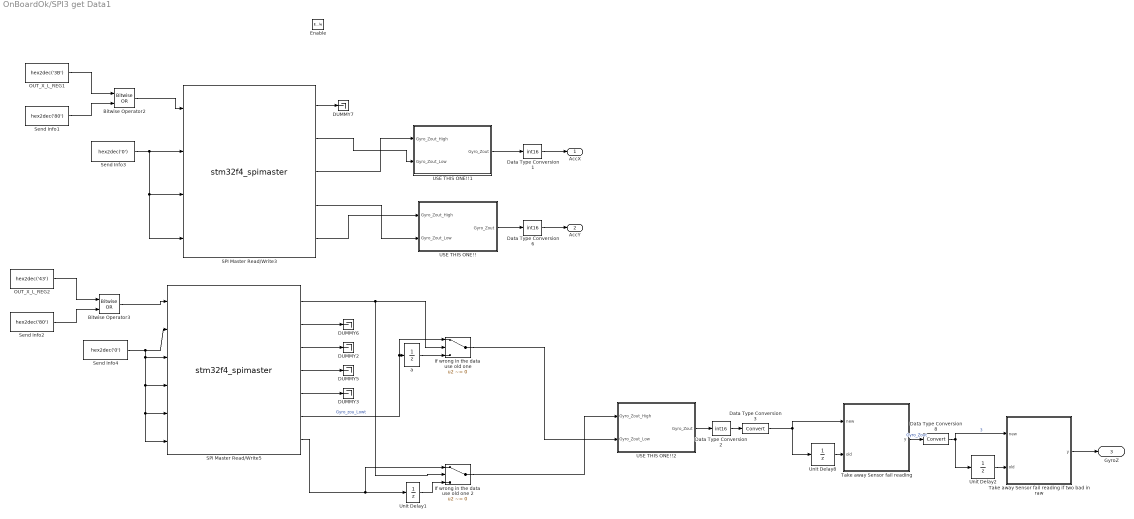
== system OnBoardOk/SPI3 get Data1 ==
  Enable : EnablePort
  " a" : UnitDelay  SampleTime=-1
  Bitwise Operator2 : simulink/Logic and Bit Operations/Bitwise Operator  logicop=OR  UseBitMask=off  NumInputPorts=2  BitMask=bin2dec('11011001')  BitMaskRealWorld=Stored Integer
  Bitwise Operator3 : simulink/Logic and Bit Operations/Bitwise Operator  logicop=OR  UseBitMask=off  NumInputPorts=2  BitMask=bin2dec('11011001')  BitMaskRealWorld=Stored Integer
  DUMMY{2..3,5..7} (5 alike) : Terminator
  Data Type Conversion1 : DataTypeConversion  OutDataTypeStr=int16
  Data Type Conversion2 : DataTypeConversion  OutDataTypeStr=int16
  Data Type Conversion3 : DataTypeConversion
  Data Type Conversion6 : DataTypeConversion  OutDataTypeStr=int16
  Data Type Conversion8 : DataTypeConversion
  If wrong in the data use old one : Switch  Criteria=u2 ~= 0
  If wrong in the data use old one 2 : Switch  Criteria=u2 ~= 0
  OUT_X_L_REG1 : Constant  Value=hex2dec('3B')  OutDataTypeStr=uint8
  OUT_X_L_REG2 : Constant  Value=hex2dec('43')  OutDataTypeStr=uint8
  SPI Master Read/Write3 : S-Function  FunctionName=stm32f4_spimaster  Parameters=mode,configuration,module,datacount,inputtypearray,outputtypearray,confstr,sampletime,sampletimestr,blockid  SFunctionDeploymentMode=off  EnableBusSupport=off  mask(stm32f4_spimaster){configuration=Transaction, module=3, mode=Read/ Write, lastmodule=1, direction=Full-Duplex, dataformat=8bit/ FirstBit_MSB, prescaler=4, cpolcpha=CPOL_Low/ CPHA_1Edge, datacount=4, nssmode=Custom, nsspin=Not used, softnssport=E, softnsspin=0, sckpin=A5, misopin=A6, mosipin=A7, inputtypearray=[4 3 3 3 3], outputtypearray=[5 7 3 3 3 3], confstr=["SPI_Direction_2Lines_FullDuplex","8b","MSB","Low","1Edge","4","Soft","0","x","x","0","x","x","1","A","5","1","A","6","1","A","7","1","0","0","0","0","0","0","0","0","PP","0","UP"], sampletime=-1, sampletimestr=Inf, blockid=SPI3getData1SPIMasterReadWrite3}
      mask prompts: module "SPI Module:"; lastmodule "Last module:"; dataformat "Data format:"; prescaler "Buad rate prescaler: Pclk/"; cpolcpha "Clock polarity (CPOL)/ Clock phase (CPHA):"; datacount "Data Read/Write count:"; nssmode "Slave/chip select (nSS, nCS) mode"; nsspin "Slave/chip select (nSS, nCS) pin"; softnssport "Slave/chip select port (nSS, nCS)"; softnsspin "Slave/chip select pin (nSS, nCS)"; sckpin "SCLK pin:"; misopin "MISO pin:"; mosipin "MOSI pin:"; inputtypearray "Input type array"; outputtypearray "Output type array"; confstr "Configuration string"; sampletime "Sample time (sec)"; sampletimestr "Compiled sample time (sec) in string"
      mask help:
      | Status:
      |  0 - Success.
      |  Otherwise - Fail.
      mask init:
      | stm32f4_spimaster_callback('init');
      mask Help: web(fullfile(waijungdocroot,'stm32f4_spimaster_readwrite.htm'), '-browser')
      mask TypeOptions configuration: Setup | Transaction
      mask Callback configuration: stm32f4_spimaster_callback('configuration');
      mask TypeOptions module: 1 | 2 | 3
      mask Callback module: stm32f4_spimaster_callback('module');
      mask TypeOptions mode: Read/ Write | Read | Write
      mask Callback mode: stm32f4_spimaster_callback('mode');
      mask TypeOptions direction: Full-Duplex | Half-Duplex_Tx | Half-Duplex_Rx
      mask Callback direction: stm32f4_spimaster_callback('direction');
      mask TypeOptions dataformat: 8bit/ FirstBit_MSB | 8bit/ FirstBit_LSB | 16bit/ FirstBit_MSB | 16bit/ FirstBit_LSB
      mask TypeOptions prescaler: 2 | 4 | 8 | 16 | 32 | 64 | 128 | 256
      mask TypeOptions cpolcpha: CPOL_Low/ CPHA_1Edge | CPOL_Low/ CPHA_2Edge | CPOL_High/ CPHA_1Edge | CPOL_High/ CPHA_2Edge
      mask Callback datacount: stm32f4_spimaster_callback('datacount');
      mask TypeOptions nssmode: Hardware | Software | Custom
      mask Callback nssmode: stm32f4_spimaster_callback('nssmode');
      mask TypeOptions nsspin: Not used | A4 | A15
      mask TypeOptions softnssport: A | B | C | D | E | F | G | H | I
      mask TypeOptions softnsspin: 0 | 1 | 2 | 3 | 4 | 5 | 6 | 7 | 8 | 9 | 10 | 11 | 12 | 13 | 14 | 15
      mask TypeOptions sckpin: Not used | A5 | B3
      mask TypeOptions misopin: Not used | A6 | B4
      mask TypeOptions mosipin: Not used | A7 | B5
      mask Callback confstr: stm32f4_spimaster_callback('confstr');
      mask Callback sampletime: stm32f4_spimaster_callback('sampletime');
      mask Callback sampletimestr: stm32f4_spimaster_callback('sampletimestr');
      mask Callback blockid: stm32f4_spimaster_callback('blockid');
      mask Display: text(0.5, 0.5, 'Module: SPI3 (Master)\nRead/ Write\nTs (sec): Inf','ver','middle','hor','center');port_label('input', 1,'Wr0 (uint8)');port_label('input', 2,'Wr1 (uint8)');port_label('input', 3,'Wr2 (uint8)');port_label('input', 4,'Wr3 (uint8)');port_label('output', 1,'Status');port_label('output', 2,'Rd0 (uint8)');port_label('output', 3,'Rd1 (uint8)');port_label('output', 4,'Rd2 (uint8)');port_label('output', 5,'Rd3 (uint8)');
  SPI Master Read/Write5 : S-Function  FunctionName=stm32f4_spimaster  Parameters=mode,configuration,module,datacount,inputtypearray,outputtypearray,confstr,sampletime,sampletimestr,blockid  SFunctionDeploymentMode=off  EnableBusSupport=off  mask(stm32f4_spimaster){configuration=Transaction, module=3, mode=Read/ Write, lastmodule=1, direction=Full-Duplex, dataformat=8bit/ FirstBit_MSB, prescaler=4, cpolcpha=CPOL_Low/ CPHA_1Edge, datacount=6, nssmode=Custom, nsspin=Not used, softnssport=E, softnsspin=0, sckpin=A5, misopin=A6, mosipin=A7, inputtypearray=[6 3 3 3 3 3 3], outputtypearray=[7 7 3 3 3 3 3 3], confstr=["SPI_Direction_2Lines_FullDuplex","8b","MSB","Low","1Edge","4","Soft","0","x","x","0","x","x","1","A","5","1","A","6","1","A","7","1","0","0","0","0","0","0","0","0","PP","0","UP"], sampletime=-1, sampletimestr=Inf, blockid=SPI3getData1SPIMasterReadWrite5}
      mask prompts: module "SPI Module:"; lastmodule "Last module:"; dataformat "Data format:"; prescaler "Buad rate prescaler: Pclk/"; cpolcpha "Clock polarity (CPOL)/ Clock phase (CPHA):"; datacount "Data Read/Write count:"; nssmode "Slave/chip select (nSS, nCS) mode"; nsspin "Slave/chip select (nSS, nCS) pin"; softnssport "Slave/chip select port (nSS, nCS)"; softnsspin "Slave/chip select pin (nSS, nCS)"; sckpin "SCLK pin:"; misopin "MISO pin:"; mosipin "MOSI pin:"; inputtypearray "Input type array"; outputtypearray "Output type array"; confstr "Configuration string"; sampletime "Sample time (sec)"; sampletimestr "Compiled sample time (sec) in string"
      mask help:
      | Status:
      |  0 - Success.
      |  Otherwise - Fail.
      mask init:
      | stm32f4_spimaster_callback('init');
      mask Help: web(fullfile(waijungdocroot,'stm32f4_spimaster_readwrite.htm'), '-browser')
      mask TypeOptions configuration: Setup | Transaction
      mask Callback configuration: stm32f4_spimaster_callback('configuration');
      mask TypeOptions module: 1 | 2 | 3
      mask Callback module: stm32f4_spimaster_callback('module');
      mask TypeOptions mode: Read/ Write | Read | Write
      mask Callback mode: stm32f4_spimaster_callback('mode');
      mask TypeOptions direction: Full-Duplex | Half-Duplex_Tx | Half-Duplex_Rx
      mask Callback direction: stm32f4_spimaster_callback('direction');
      mask TypeOptions dataformat: 8bit/ FirstBit_MSB | 8bit/ FirstBit_LSB | 16bit/ FirstBit_MSB | 16bit/ FirstBit_LSB
      mask TypeOptions prescaler: 2 | 4 | 8 | 16 | 32 | 64 | 128 | 256
      mask TypeOptions cpolcpha: CPOL_Low/ CPHA_1Edge | CPOL_Low/ CPHA_2Edge | CPOL_High/ CPHA_1Edge | CPOL_High/ CPHA_2Edge
      mask Callback datacount: stm32f4_spimaster_callback('datacount');
      mask TypeOptions nssmode: Hardware | Software | Custom
      mask Callback nssmode: stm32f4_spimaster_callback('nssmode');
      mask TypeOptions nsspin: Not used | A4 | A15
      mask TypeOptions softnssport: A | B | C | D | E | F | G | H | I
      mask TypeOptions softnsspin: 0 | 1 | 2 | 3 | 4 | 5 | 6 | 7 | 8 | 9 | 10 | 11 | 12 | 13 | 14 | 15
      mask TypeOptions sckpin: Not used | A5 | B3
      mask TypeOptions misopin: Not used | A6 | B4
      mask TypeOptions mosipin: Not used | A7 | B5
      mask Callback confstr: stm32f4_spimaster_callback('confstr');
      mask Callback sampletime: stm32f4_spimaster_callback('sampletime');
      mask Callback sampletimestr: stm32f4_spimaster_callback('sampletimestr');
      mask Callback blockid: stm32f4_spimaster_callback('blockid');
      mask Display: text(0.5, 0.5, 'Module: SPI3 (Master)\nRead/ Write\nTs (sec): Inf','ver','middle','hor','center');port_label('input', 1,'Wr0 (uint8)');port_label('input', 2,'Wr1 (uint8)');port_label('input', 3,'Wr2 (uint8)');port_label('input', 4,'Wr3 (uint8)');port_label('input', 5,'Wr4 (uint8)');port_label('input', 6,'Wr5 (uint8)');port_label('output', 1,'Status');port_label('output', 2,'Rd0 (uint8)');port_label('output', 3,'Rd1 (uint8)');port_label('output', 4,'Rd2 (uint8)');port_label('output', 5,'Rd3 (uint8)');port_label('output', 6,'Rd4 (uint8)');port_label('output', 7,'Rd5 (uint8)');
  Send Info1 : Constant  Value=hex2dec('80')  OutDataTypeStr=uint8
  Send Info2 : Constant  Value=hex2dec('80')  OutDataTypeStr=uint8
  Send Info3 : Constant  Value=hex2dec('0')  OutDataTypeStr=uint8
  Send Info4 : Constant  Value=hex2dec('0')  OutDataTypeStr=uint8
  Take away Sensor fail reading : MATLAB Function  TreatAsAtomicUnit=on
  Take away Sensor fail reading if two bad in raw : MATLAB Function  TreatAsAtomicUnit=on
  USE THIS ONE!! : Subsystem
  USE THIS ONE!!1 : Subsystem
  USE THIS ONE!!2 : Subsystem
  Unit Delay1 : UnitDelay  SampleTime=-1
  Unit Delay2 : UnitDelay  InitialCondition=-40.45  SampleTime=-1
  Unit Delay8 : UnitDelay  InitialCondition=-40.45  SampleTime=-1
  AccX : Outport
  "AccY " : Outport  Port=2
  GyroZ : Outport  Port=3
  wires:
  SPI Master Read/Write5/2 -> DUMMY6/1
  SPI Master Read/Write5/4 -> DUMMY5/1
  Bitwise Operator3/1 -> SPI Master Read/Write5/1
  OUT_X_L_REG1/1 -> Bitwise Operator2/1
  OUT_X_L_REG2/1 -> Bitwise Operator3/1
  Send Info2/1 -> Bitwise Operator3/2
  Bitwise Operator2/1 -> SPI Master Read/Write3/1
  Send Info3/1 -> SPI Master Read/Write3/4, SPI Master Read/Write3/3, SPI Master Read/Write3/2
  Send Info1/1 -> Bitwise Operator2/2
  Send Info4/1 -> SPI Master Read/Write5/6, SPI Master Read/Write5/5, SPI Master Read/Write5/4, SPI Master Read/Write5/3, SPI Master Read/Write5/2
  SPI Master Read/Write3/1 -> DUMMY7/1
  SPI Master Read/Write5/3 -> DUMMY2/1
  SPI Master Read/Write5/5 -> DUMMY3/1
  SPI Master Read/Write3/2 -> USE THIS ONE!!1/2(Gyro_Zout_Low)
  SPI Master Read/Write3/3 -> USE THIS ONE!!1/1("Gyro_Zout_High ")
  SPI Master Read/Write3/4 -> USE THIS ONE!!/2(Gyro_Zout_Low)
  SPI Master Read/Write3/5 -> USE THIS ONE!!/1("Gyro_Zout_High ")
  USE THIS ONE!!1/1(Gyro_Zout) -> Data Type Conversion1/1
  USE THIS ONE!!/1(Gyro_Zout) -> Data Type Conversion6/1
  Data Type Conversion6/1 -> "AccY "/1
  Data Type Conversion1/1 -> AccX/1
  USE THIS ONE!!2/1(Gyro_Zout) -> Data Type Conversion2/1
  Data Type Conversion2/1 -> Data Type Conversion3/1
  SPI Master Read/Write5/6 -> " a"/1, If wrong in the data use old one/1  "Gyro_zou_Lowt"
  " a"/1 -> If wrong in the data use old one/3
  SPI Master Read/Write5/7 -> If wrong in the data use old one 2/1, Unit Delay1/1
  SPI Master Read/Write5/1 -> If wrong in the data use old one 2/2, If wrong in the data use old one/2
  Unit Delay1/1 -> If wrong in the data use old one 2/3
  If wrong in the data use old one/1 -> USE THIS ONE!!2/2(Gyro_Zout_Low)
  If wrong in the data use old one 2/1 -> USE THIS ONE!!2/1("Gyro_Zout_High ")
  Unit Delay8/1 -> Take away Sensor fail reading/2(old)
  Take away Sensor fail reading/1(y) -> Data Type Conversion8/1  "Gyro_Zout"
  Unit Delay2/1 -> Take away Sensor fail reading if two bad in raw/2(old)
  Data Type Conversion8/1 -> Unit Delay2/1, Take away Sensor fail reading if two bad in raw/1(new)  "3"
  Take away Sensor fail reading if two bad in raw/1(y) -> GyroZ/1
  Data Type Conversion3/1 -> Unit Delay8/1, Take away Sensor fail reading/1(new)

== system OnBoardOk/Start Callibration2 ==
  Trigger : TriggerPort  PortDimensions=1
  Constant2 : Constant
  Start Callibration : Outport  InitialOutput=[0]
  wires:
  Constant2/1 -> Start Callibration/1

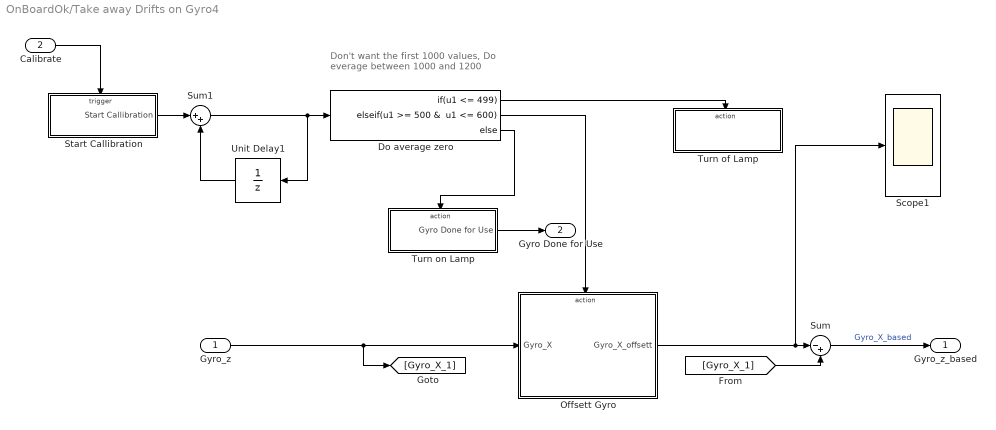
== system OnBoardOk/Take away Drifts on Gyro4 ==
  note: Don't want the first 1000 values,
      | Do everage between 1000 and 1200
  Gyro_z : Inport
  Calibrate : Inport  Port=2
  Do average zero : If  IfExpression=u1 <= 499  ElseIfExpressions="u1 >= 500 &  u1 <= 600"
  Offsett Gyro : Subsystem
  Scope1 : Scope
  Start Callibration : Subsystem
  Sum : Sum  Inputs=|-+
  Sum1 : Sum  Inputs=|++
  Turn of Lamp : Subsystem
  Turn on Lamp : Subsystem
  Unit Delay1 : UnitDelay  SampleTime=-1
  Gyro_z_based : Outport
  Gyro Done for Use : Outport  Port=2
  wires:
  Unit Delay1/1 -> Sum1/2
  Sum1/1 -> Do average zero/1, Unit Delay1/1
  [Gyro_X_1] -> Sum/2
  Offsett Gyro/1(Gyro_X_offsett) -> Scope1/1, Sum/1
  Sum/1 -> Gyro_z_based/1  "Gyro_X_based"
  Gyro_z/1 -> [Gyro_X_1], Offsett Gyro/1(Gyro_X)
  Do average zero/2 -> Offsett Gyro/Action
  Do average zero/3 -> Turn on Lamp/Action
  Calibrate/1 -> Start Callibration/Trigger
  Start Callibration/1(Start Callibration) -> Sum1/1
  Do average zero/1 -> Turn of Lamp/Action
  Turn on Lamp/1(Gyro Done for Use) -> Gyro Done for Use/1
